simulink library "SLlib_lka_thesis"  (R2018a)
settings: Solver=ode45  StartTime=0.0  StopTime=10.0  RelTol=1e-3  EnableMultiTasking=on
undefined symbols (not defined in the file or in its folder): contr, curvature, DiscIntNeverNeededParam, k, l, pin, sysCtrl
libraries: $bdroot x16, cstblocks x1, simulink x1
(part 1 of 2)
settings Model: Creator=Georg  LastModifiedBy=georgnestlinger
settings DataIOCC: LimitDataPoints=on  SaveFormat=Array  SignalLoggingSaveFormat=ModelDataLogs
settings OptimizationCC: ExpressionDepthLimit=2147483647  LifeSpan=inf
settings DebuggingCC: UnderspecifiedInitializationDetection=Classic  MergeDetectMultiDrivingBlocksExec=none  SolverPrmCheckMsg=warning  FcnCallInpInsideContextMsg=warning  StateNameClashWarn=warning  SFUnexpectedBacktrackingDiag=warning  SFNoUnconditionalDefaultTransitionDiag=warning  SFExecutionAtInitializationDiag=none
settings HardwareCC: ProdBitPerPointer=32  ProdBitPerSizeT=32  ProdBitPerPtrDiffT=32  ProdLargestAtomicFloat=None  ProdIntDivRoundTo=Undefined  ProdEndianess=Unspecified  ProdWordSize=32  ProdHWDeviceType=32-bit Generic
settings ModelReferenceCC: PropagateSignalLabelsOutOfModel=off
settings CodeAppCC: StateflowObjectComments=on
settings GRTTargetCC: TargetLangStandard=C89/C90 (ANSI)  GeneratePreprocessorConditionals=Disable all  CombineOutputUpdateFcns=off  GRTInterface=on
settings ConfigComp: CovMetricSettings=dw  CovHtmlReporting=on  CovSaveCumulativeToWorkspaceVar=on  CovSaveSingleToWorkspaceVar=on  CovExternalEMLEnable=off

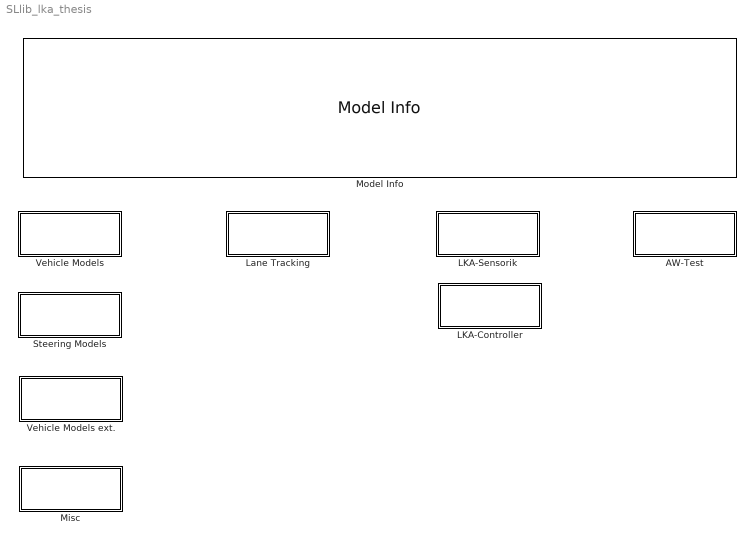
== system SLlib_lka_thesis ==
  AW-Test : Subsystem
  LKA-Controller : Subsystem
  LKA-Sensorik : Subsystem
  Lane Tracking : Subsystem
  Misc : Subsystem
  Model Info : simulink/Model-Wide Utilities/Model Info  Frame=on  DisplayStringWithTags=|  HorizontalTextAlignment=Left  LeftAlignmentValue=0.02
      | Author: Georg Nestlinger
      | Master thesis: Modellbildung und Simulation eines Spurhalteassistenzsystems 
      | 
      | Created: %<Created>
      | 
      | ModifiedBy: %<ModifiedBy>
      | ModifiedComment: %<ModifiedComment>
      | 
      | ModelVersion: %<ModelVersion>
      | ModelName: %<ModelName>
      | 
      | LastModifiedBy: %<LastModifiedBy>
      | LastModidifiedDate: %<LastModificationDate>
  Steering Models : Subsystem
  Vehicle Models : Subsystem
  Vehicle Models ext. : Subsystem

== system SLlib_lka_thesis/AW-Test ==
  AW-Loop : Subsystem
  Plot Interface : Subsystem

== system SLlib_lka_thesis/LKA-Controller ==
  AlgSynth : Subsystem
  FKL : Subsystem
  LKA-Controller : Subsystem  BlockChoice=LQR_2int
      settings: TemplateBlock=self  MemberBlocks=AlgSynth,FKL,LQR,LQR_2int,ZR,ZR_2int
  LQR : Subsystem
  LQR_2int : Subsystem
  State Feedback : Subsystem  TreatAsAtomicUnit=on  mask{fdbk=0}
      mask prompts: fdbk "Feedback parameter:"
  ZR : Subsystem
  ZR_2int : Subsystem

== system SLlib_lka_thesis/LKA-Sensorik ==
  epsL_Sensor : Subsystem
  epsL_exactMdl : Subsystem
  epsL_linMdl : Subsystem
  select epsL : Subsystem  BlockChoice=epsL_Sensor
      settings: TemplateBlock=self  MemberBlocks=epsL_Sensor,epsL_exactMdl,epsL_linMdl
  select yL : Subsystem  BlockChoice=yL_Sensor
      settings: TemplateBlock=self  MemberBlocks=yL_Sensor,yL_exactMdl,yL_linMdl
  yL_Sensor : Subsystem
  yL_exactMdl : Subsystem
  yL_linMdl : Subsystem

== system SLlib_lka_thesis/Lane Tracking ==
  Lane Tracking Model (linear&nonlinear) : Subsystem
  Lane Tracking Model (linear) : Subsystem
  Lane Tracking Model (nonlinear) : Subsystem
  Lane Tracking Sensor : Subsystem

== system SLlib_lka_thesis/Misc ==
  Simout : Subsystem

== system SLlib_lka_thesis/Steering Models ==
  Steering Model (CarMaker DSR) : Subsystem
  Steering Model (CarMaker DSR) [masked] : Subsystem  mask(Steering model parameterization){d_rot=0, d_rack=0, i=0, I_rot=0, m_left=0, m_right=0, m_rack=0, V=0, x0=[0;0]}
      mask prompts: d_rot "d_rot [Nm*s/rad]"; d_rack "d_rack [N*s/rad]"; i "i [rad/m]"; I_rot "I_rot [kg*m²]"; m_left "m_left [kg]"; m_right "m_right [kg]"; m_rack "m_rack [kg]"; V "V [-]"; x0 "Initial value [SWAngle(0); SWRate(0)]"
      mask help:
      | Enter parameters of steering model 'CarMaker Dynamic Steer Ratio'.
      | This model is taken from 'CarMaker Reference Manual, Version 4.0, p. 140'.

== system SLlib_lka_thesis/Vehicle Models ==
  Single Track Models : Subsystem

== system SLlib_lka_thesis/Vehicle Models ext. ==
  Single Track Model (linear) [Initial Values; Interface] : Subsystem
  Single Track Model (linear) [Initial Values; masked] : Subsystem  mask(Linear Single Track Model Inital Values){sy=0, vy=0, yawAngle=0, yawRate=0, x_global=0, y_global=0, s_global=0}
      mask help: Specify initial values for the linear single track model.
  Single Track Model (linear) [Parameter; Interface] : Subsystem
  Single Track Model (linear) [Parameter; masked] : Subsystem  mask(Linear Single Track Model Parameter){cs_front=0, cs_rear=0, l_front=0, l_rear=0, m=0, Izz=0}
      mask prompts: cs_front "Cornering stiffness front [N/rad]"; cs_rear "Cornering stiffness rear [N/rad]"; l_front "Distance COG - front axle [m]"; l_rear "Distance COG - rear axle [m]"; m "Vehicle mass [kg]"; Izz "Moment of inertia of yaw axis [kg*m²]"
      mask help: Specify parameters for the linear single track model.
  Single Track Model/Lane Tracking : Subsystem
  Single Track Model/Lane Tracking/Steering Model : Subsystem
  Single Track Model/Steering Model : Subsystem
  Steering Model (CarMaker DSR) [Parameter; masked] : Subsystem  mask(Steering Model Parameter: Dynamic Steer Ratio){d_rot=0, d_rack=0, i_HR=0, I_rot=0, m_left=0, m_right=0, m_rack=0, V=0, alpha=0}
      mask prompts: d_rot "Damping coefficient of rotating parts [Nm*s/rad]"; d_rack "Damping coefficient of steering rack [Ns/m]"; i_HR "Steering gear ratio steering wheel angle/rack travel [rad/m]"; I_rot "Steering inertia of all rotating parts [kg*m²]"; m_left "Left wheel suspension mass [kg]"; m_right "Right wheel suspension mass [kg]"; m_rack "Steering rack mass [kg]"; V "Amplification of the steering torque [-]"; alpha "Ratio steering wheel angle/front wheel angle [-]"
      mask help: Specify parameters for the CarMaker steering model Dynamic Steer Ratio (DSR).

== system SLlib_lka_thesis/AW-Test/AW-Loop ==
  uPlant : Inport
  delta : Inport  Port=2
  1-D Lookup Table : Lookup_n-D  NumberOfTableDimensions=1  BreakpointsForDimension1=length  Table=curvature  RndMeth=Simplest  InputSameDT=on
  Bus Selector : BusSelector  OutputSignals=vy,yawRate,latOff_LAD_nonlinear,angDev_LAD_nonlinear,SWAngle,SWRate
  Bus Selector1 : BusSelector  OutputSignals=s_global
  Gain2 : Gain  Gain=0
  Regler : Subsystem
  Sum : Sum  Inputs=|-|
  Vehicle Model : Subsystem
  States : Outport
  uCtrl : Outport  Port=2
  wires:
  Vehicle Model/1(VehicleStates) -> Bus Selector1/1, Bus Selector/1, States/1
  Regler/1(u) -> uCtrl/1
  uPlant/1 -> Sum/1
  Bus Selector/1 -> Regler/2(s_yDot)  "<vy>"
  Bus Selector/2 -> Regler/3(psiDot)  "<yawRate>"
  Bus Selector/3 -> Regler/4(yL)  "<latOff_LAD_nonlinear>"
  Bus Selector/4 -> Regler/5(epsL)  "<angDev_LAD_nonlinear>"
  Bus Selector/5 -> Regler/6(steering wheel angle)  "<SWAngle>"
  Bus Selector/6 -> Regler/7(steering wheel angle velocity)  "<SWRate>"
  Sum/1 -> Vehicle Model/1(SWTorque [Nm])
  1-D Lookup Table/1 -> Vehicle Model/3(curvature_LAD [1/m]), Gain2/1
  Bus Selector1/1 -> 1-D Lookup Table/1  "<s_global>"
  Gain2/1 -> Vehicle Model/2(F_left [N])
  delta/1 -> Regler/1(delta)

== system SLlib_lka_thesis/AW-Test/Plot Interface ==
  ideal : Inport
  mit AW : Inport  Port=2
  ohne AW : Inport  Port=3
  Gain : Gain
  Gain1 : Gain
  Gain2 : Gain
  Out1 : Outport
  Out2 : Outport  Port=2
  Out3 : Outport  Port=3
  wires:
  ideal/1 -> Gain/1
  mit AW/1 -> Gain1/1
  ohne AW/1 -> Gain2/1
  Gain/1 -> Out1/1  "ideal"
  Gain1/1 -> Out2/1  "mit AW"
  Gain2/1 -> Out3/1  "ohne AW"

== system SLlib_lka_thesis/LKA-Controller/AlgSynth ==
  r : Inport
  vy : Inport  Port=2
  psiDot : Inport  Port=3
  yL : Inport  Port=4
  epsL : Inport  Port=5
  Controller : Subsystem
  Terminator : Terminator
  Terminator1 : Terminator
  Terminator2 : Terminator
  delta [rad] : Outport
  wires:
  epsL/1 -> Terminator2/1
  vy/1 -> Terminator/1
  psiDot/1 -> Terminator1/1
  yL/1 -> Controller/2(y)
  r/1 -> Controller/1(r)
  Controller/1(u) -> delta [rad]/1

== system SLlib_lka_thesis/LKA-Controller/FKL ==
  r : Inport
  vy : Inport  Port=2
  psiDot : Inport  Port=3
  yL : Inport  Port=4
  epsL : Inport  Port=5
  LTI System R : cstblocks/LTI System  sys=contr.s.AlgSynth.R  IC=[]
  Terminator{1..4} (4 alike) : Terminator
  delta [rad] : Outport
  wires:
  epsL/1 -> Terminator3/1
  vy/1 -> Terminator1/1
  psiDot/1 -> Terminator2/1
  yL/1 -> LTI System R/1
  LTI System R/1 -> delta [rad]/1
  r/1 -> Terminator4/1

== system SLlib_lka_thesis/LKA-Controller/LKA-Controller ==
  r : Inport
  vy : Inport  Port=2
  psiDot : Inport  Port=3
  yL : Inport  Port=4
  epsL : Inport  Port=5
  LQR_2int : $bdroot/LKA-Controller/LQR_2int
  delta [rad] : Outport
  wires:
  r/1 -> LQR_2int/1
  vy/1 -> LQR_2int/2
  psiDot/1 -> LQR_2int/3
  yL/1 -> LQR_2int/4
  epsL/1 -> LQR_2int/5
  LQR_2int/1 -> delta [rad]/1

== system SLlib_lka_thesis/LKA-Controller/LQR ==
  r : Inport
  vy : Inport  Port=2
  psiDot : Inport  Port=3
  yL : Inport  Port=4
  epsL : Inport  Port=5
  Gain1 : Gain  Gain=-contr.t.LQR.k  Multiplication=Matrix(K*u) (u vector)
  Mux : Mux
  Sum1 : Sum  Inputs=-+|
  delta [rad] : Outport
  wires:
  Gain1/1 -> delta [rad]/1
  Mux/1 -> Gain1/1
  epsL/1 -> Mux/4
  vy/1 -> Mux/1
  psiDot/1 -> Mux/2
  yL/1 -> Sum1/2
  Sum1/1 -> Mux/3
  r/1 -> Sum1/1

== system SLlib_lka_thesis/LKA-Controller/LQR_2int ==
  r : Inport
  vy : Inport  Port=2
  psiDot : Inport  Port=3
  yL : Inport  Port=4
  epsL : Inport  Port=5
  Gain : Gain  Gain=-contr.t.LQR_2int.k  Multiplication=Matrix(K*u) (u vector)
  Integrator2 : Integrator
  Integrator3 : Integrator
  Mux2 : Mux  Inputs=6
  Sum1 : Sum  Inputs=-+|
  delta [rad] : Outport
  wires:
  Mux2/1 -> Gain/1
  epsL/1 -> Mux2/4
  vy/1 -> Mux2/1
  psiDot/1 -> Mux2/2
  yL/1 -> Sum1/2
  Sum1/1 -> Mux2/3, Integrator2/1
  r/1 -> Sum1/1
  Integrator2/1 -> Mux2/6, Integrator3/1
  Integrator3/1 -> Mux2/5
  Gain/1 -> delta [rad]/1

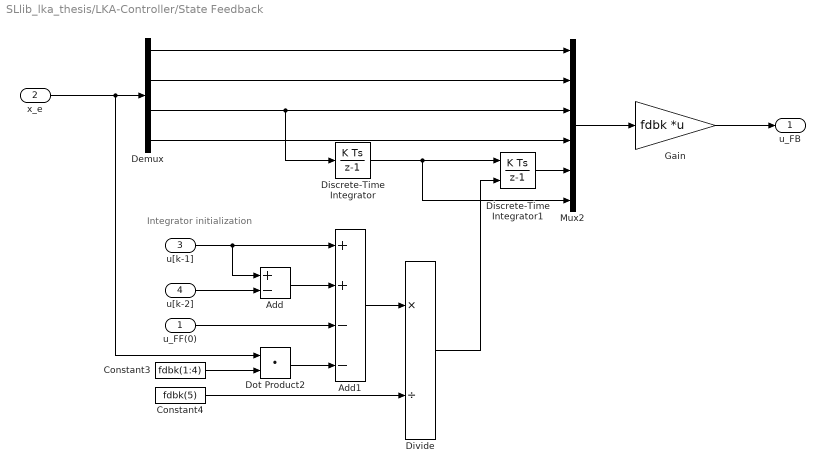
== system SLlib_lka_thesis/LKA-Controller/State Feedback ==
  note: Integrator initialization
  u_FF(0) : Inport
  x_e : Inport  Port=2
  u[k-1] : Inport  Port=3
  u[k-2] : Inport  Port=4
  Add : Sum  Inputs=+-
  Add1 : Sum  Inputs=++--
  Constant3 : Constant  Value=fdbk(1:4)
  Constant4 : Constant  Value=fdbk(5)
  Demux : Demux
  Discrete-Time Integrator : DiscreteIntegrator  SampleTime=-1  ICPrevOutput=DiscIntNeverNeededParam  ICPrevScaledInput=DiscIntNeverNeededParam
  Discrete-Time Integrator1 : DiscreteIntegrator  InitialConditionSource=external  SampleTime=-1  ICPrevOutput=DiscIntNeverNeededParam  ICPrevScaledInput=DiscIntNeverNeededParam
  Divide : Product  Inputs=*/
  Dot Product2 : DotProduct  InputSameDT=on  OutDataTypeStr=Inherit: Inherit via internal rule
  Gain : Gain  Gain=fdbk  Multiplication=Matrix(K*u) (u vector)
  Mux2 : Mux  Inputs=6
  u_FB : Outport
  wires:
  u[k-2]/1 -> Add/2
  Demux/1 -> Mux2/1
  Divide/1 -> Discrete-Time Integrator1/2
  x_e/1 -> Dot Product2/1, Demux/1
  Add1/1 -> Divide/1
  Demux/2 -> Mux2/2
  Mux2/1 -> Gain/1
  u[k-1]/1 -> Add/1, Add1/1
  Demux/3 -> Discrete-Time Integrator/1, Mux2/3
  Constant4/1 -> Divide/2
  Constant3/1 -> Dot Product2/2
  Demux/4 -> Mux2/4
  Discrete-Time Integrator1/1 -> Mux2/5
  Gain/1 -> u_FB/1
  Discrete-Time Integrator/1 -> Discrete-Time Integrator1/1, Mux2/6
  Dot Product2/1 -> Add1/4
  u_FF(0)/1 -> Add1/3
  Add/1 -> Add1/2

== system SLlib_lka_thesis/LKA-Controller/ZR ==
  r : Inport
  vy : Inport  Port=2
  psiDot : Inport  Port=3
  yL : Inport  Port=4
  epsL : Inport  Port=5
  Gain1 : Gain  Gain=-contr.t.ZR.k  Multiplication=Matrix(K*u) (u vector)
  Mux : Mux
  Sum1 : Sum  Inputs=-+|
  delta [rad] : Outport
  wires:
  Gain1/1 -> delta [rad]/1
  Mux/1 -> Gain1/1
  epsL/1 -> Mux/4
  vy/1 -> Mux/1
  psiDot/1 -> Mux/2
  yL/1 -> Sum1/2
  Sum1/1 -> Mux/3
  r/1 -> Sum1/1

== system SLlib_lka_thesis/LKA-Controller/ZR_2int ==
  r : Inport
  vy : Inport  Port=2
  psiDot : Inport  Port=3
  yL : Inport  Port=4
  epsL : Inport  Port=5
  Gain1 : Gain  Gain=-contr.t.ZR_2int.k  Multiplication=Matrix(K*u) (u vector)
  Integrator2 : Integrator
  Integrator3 : Integrator
  Mux2 : Mux  Inputs=6
  Sum1 : Sum  Inputs=-+|
  delta [rad] : Outport
  wires:
  Mux2/1 -> Gain1/1
  epsL/1 -> Mux2/4
  vy/1 -> Mux2/1
  psiDot/1 -> Mux2/2
  yL/1 -> Sum1/2
  Sum1/1 -> Mux2/3, Integrator2/1
  r/1 -> Sum1/1
  Integrator2/1 -> Mux2/6, Integrator3/1
  Integrator3/1 -> Mux2/5
  Gain1/1 -> delta [rad]/1

== system SLlib_lka_thesis/LKA-Sensorik/epsL_Sensor ==
  Vehicle_Data : Inport
  Bus Selector8 : BusSelector  OutputSignals=Sensor.angularDev_LAD_Sensor
  epsL : Outport
  wires:
  Vehicle_Data/1 -> Bus Selector8/1
  Bus Selector8/1 -> epsL/1  "<angularDev_LAD_Sensor>"

== system SLlib_lka_thesis/LKA-Sensorik/epsL_exactMdl ==
  Vehicle_Data : Inport
  Bus Selector8 : BusSelector  OutputSignals=VehicleState.angularDev_LAD_nonlinear
  epsL : Outport
  wires:
  Vehicle_Data/1 -> Bus Selector8/1
  Bus Selector8/1 -> epsL/1  "<angularDev_LAD_nonlinear>"

== system SLlib_lka_thesis/LKA-Sensorik/epsL_linMdl ==
  Vehicle_Data : Inport
  Bus Selector8 : BusSelector  OutputSignals=VehicleState.angularDev_LAD_linear
  epsL : Outport
  wires:
  Vehicle_Data/1 -> Bus Selector8/1
  Bus Selector8/1 -> epsL/1  "<angularDev_LAD_linear>"

== system SLlib_lka_thesis/LKA-Sensorik/select epsL ==
  Vehicle_Data : Inport
  epsL_Sensor : $bdroot/LKA-Sensorik/epsL_Sensor
  epsL : Outport
  wires:
  Vehicle_Data/1 -> epsL_Sensor/1
  epsL_Sensor/1 -> epsL/1

== system SLlib_lka_thesis/LKA-Sensorik/select yL ==
  Vehicle_Data : Inport
  yL_Sensor : $bdroot/LKA-Sensorik/yL_Sensor
  yL : Outport
  wires:
  Vehicle_Data/1 -> yL_Sensor/1
  yL_Sensor/1 -> yL/1

== system SLlib_lka_thesis/LKA-Sensorik/yL_Sensor ==
  Vehicle_Data : Inport
  Bus Selector8 : BusSelector  OutputSignals=Sensor.lateralOff_LAD_Sensor
  yL : Outport
  wires:
  Vehicle_Data/1 -> Bus Selector8/1
  Bus Selector8/1 -> yL/1  "<lateralOff_LAD_Sensor>"

== system SLlib_lka_thesis/LKA-Sensorik/yL_exactMdl ==
  Vehicle_Data : Inport
  Bus Selector8 : BusSelector  OutputSignals=VehicleState.lateralOff_LAD_nonlinear
  yL : Outport
  wires:
  Bus Selector8/1 -> yL/1  "<lateralOff_LAD_nonlinear>"
  Vehicle_Data/1 -> Bus Selector8/1

== system SLlib_lka_thesis/LKA-Sensorik/yL_linMdl ==
  Vehicle_Data : Inport
  Bus Selector1 : BusSelector  OutputSignals=VehicleState.lateralOff_LAD_linear
  yL : Outport
  wires:
  Vehicle_Data/1 -> Bus Selector1/1
  Bus Selector1/1 -> yL/1  "<lateralOff_LAD_linear>"

== system SLlib_lka_thesis/Lane Tracking/Lane Tracking Model (linear&nonlinear) ==
  vx [m/s] : Inport  OutDataTypeStr=double  PortDimensions=1
  vy [m/s] : Inport  Port=2  OutDataTypeStr=double  PortDimensions=1
  yawRate [rad/s] : Inport  Port=3  OutDataTypeStr=double  PortDimensions=1
  LAD [m] : Inport  Port=4  OutDataTypeStr=double  PortDimensions=1
  curvature_LAD [1/m] : Inport  Port=5  OutDataTypeStr=double  PortDimensions=1
  lateralOff_LAD(0) [m] : Inport  Port=6  OutDataTypeStr=double  PortDimensions=1
  angularDev_LAD(0) [rad] : Inport  Port=7  OutDataTypeStr=double  PortDimensions=1
  Bus Creator : BusCreator  Inputs=4
  Lane Tracking Model (linear) : $bdroot/Lane Tracking/Lane Tracking Model (linear)
  Lane Tracking Model (nonlinear) : $bdroot/Lane Tracking/Lane Tracking Model (nonlinear)
  LaneTracking : Outport
  wires:
  vx [m/s]/1 -> Lane Tracking Model (linear)/1, Lane Tracking Model (nonlinear)/1
  vy [m/s]/1 -> Lane Tracking Model (linear)/2, Lane Tracking Model (nonlinear)/2
  yawRate [rad/s]/1 -> Lane Tracking Model (linear)/3, Lane Tracking Model (nonlinear)/3
  LAD [m]/1 -> Lane Tracking Model (linear)/4, Lane Tracking Model (nonlinear)/4
  curvature_LAD [1/m]/1 -> Lane Tracking Model (linear)/5, Lane Tracking Model (nonlinear)/5
  lateralOff_LAD(0) [m]/1 -> Lane Tracking Model (linear)/6, Lane Tracking Model (nonlinear)/6
  angularDev_LAD(0) [rad]/1 -> Lane Tracking Model (linear)/7, Lane Tracking Model (nonlinear)/7
  Bus Creator/1 -> LaneTracking/1  "LaneTracking"
  Lane Tracking Model (linear)/1 -> Bus Creator/1
  Lane Tracking Model (nonlinear)/2 -> Bus Creator/4
  Lane Tracking Model (linear)/2 -> Bus Creator/2
  Lane Tracking Model (nonlinear)/1 -> Bus Creator/3

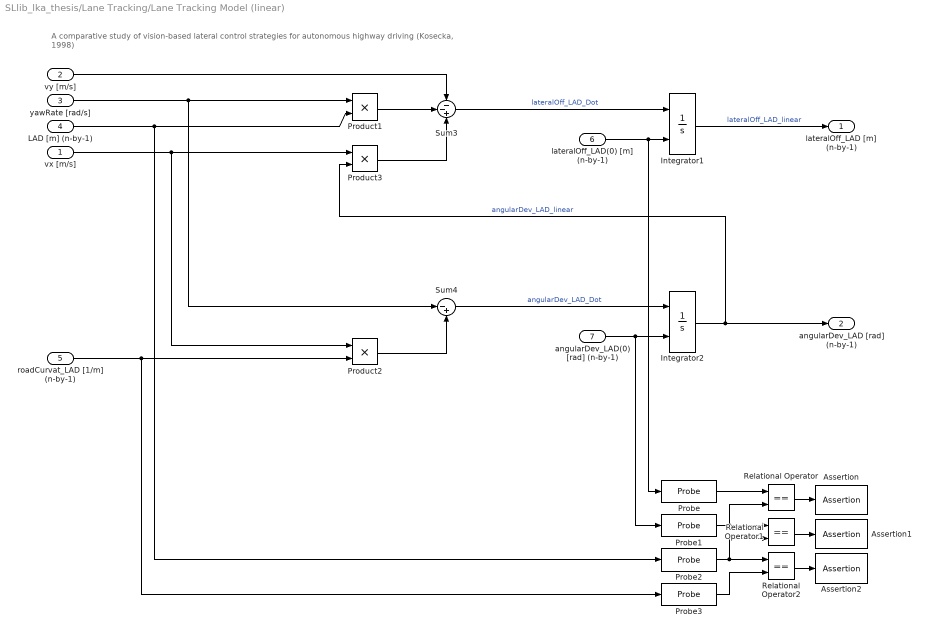
== system SLlib_lka_thesis/Lane Tracking/Lane Tracking Model (linear) ==
  note: A comparative study of vision-based lateral control strategies for autonomous highway driving (Kosecka, 1998)
  vx [m/s] : Inport  OutDataTypeStr=double  Unit=m/s  PortDimensions=1
  vy [m/s] : Inport  Port=2  OutDataTypeStr=double  Unit=m/s  PortDimensions=1
  yawRate [rad/s] : Inport  Port=3  OutDataTypeStr=double  Unit=rad/s  PortDimensions=1
  LAD [m] (n-by-1) : Inport  Port=4  OutDataTypeStr=double  Unit=m
  roadCurvat_LAD [1/m] (n-by-1) : Inport  Port=5  OutDataTypeStr=double  Unit=1/m
  lateralOff_LAD(0) [m] (n-by-1) : Inport  Port=6  OutDataTypeStr=double  Unit=meter
  angularDev_LAD(0) [rad] (n-by-1) : Inport  Port=7  OutDataTypeStr=double  Unit=rad
  Assertion : Assertion
  Assertion1 : Assertion
  Assertion2 : Assertion
  Integrator1 : Integrator  InitialConditionSource=external  InitialCondition=pin.VehicleModel.initialValue.yL
  Integrator2 : Integrator  InitialConditionSource=external  InitialCondition=pin.VehicleModel.initialValue.yL
  Probe{,1..3} (4 alike) : Probe  ProbeWidth=off  ProbeSampleTime=off  ProbeComplexSignal=off  ProbeSignalDimensions=on
  Product1 : Product  RndMeth=Zero
  Product2 : Product  RndMeth=Zero
  Product3 : Product  RndMeth=Zero
  Relational Operator : RelationalOperator  Operator===  OutDataTypeStr=boolean  RndMeth=Nearest
  Relational Operator1 : RelationalOperator  Operator===  OutDataTypeStr=boolean  RndMeth=Nearest
  Relational Operator2 : RelationalOperator  Operator===  OutDataTypeStr=boolean  RndMeth=Nearest
  Sum3 : Sum  Inputs=--+
  Sum4 : Sum  Inputs=|-+
  lateralOff_LAD [m] (n-by-1) : Outport  OutDataTypeStr=double  Unit=m
  angularDev_LAD [rad] (n-by-1) : Outport  Port=2  OutDataTypeStr=double  Unit=rad
  wires:
  roadCurvat_LAD [1/m] (n-by-1)/1 -> Product2/2, Probe3/1
  Integrator1/1 -> lateralOff_LAD [m] (n-by-1)/1  "lateralOff_LAD_linear"
  yawRate [rad/s]/1 -> Product1/1, Sum4/1
  vy [m/s]/1 -> Sum3/1
  Integrator2/1 -> angularDev_LAD [rad] (n-by-1)/1, Product3/2  "angularDev_LAD_linear"
  Product3/1 -> Sum3/3
  Sum3/1 -> Integrator1/1  "lateralOff_LAD_Dot"
  Sum4/1 -> Integrator2/1  "angularDev_LAD_Dot"
  Product2/1 -> Sum4/2
  vx [m/s]/1 -> Product2/1, Product3/1
  LAD [m] (n-by-1)/1 -> Product1/2, Probe2/1
  Product1/1 -> Sum3/2
  angularDev_LAD(0) [rad] (n-by-1)/1 -> Integrator2/2, Probe1/1
  lateralOff_LAD(0) [m] (n-by-1)/1 -> Integrator1/2, Probe/1
  Probe/1 -> Relational Operator/1
  Relational Operator/1 -> Assertion/1
  Relational Operator1/1 -> Assertion1/1
  Relational Operator2/1 -> Assertion2/1
  Probe1/1 -> Relational Operator1/1, Relational Operator/2
  Probe2/1 -> Relational Operator2/1, Relational Operator1/2
  Probe3/1 -> Relational Operator2/2

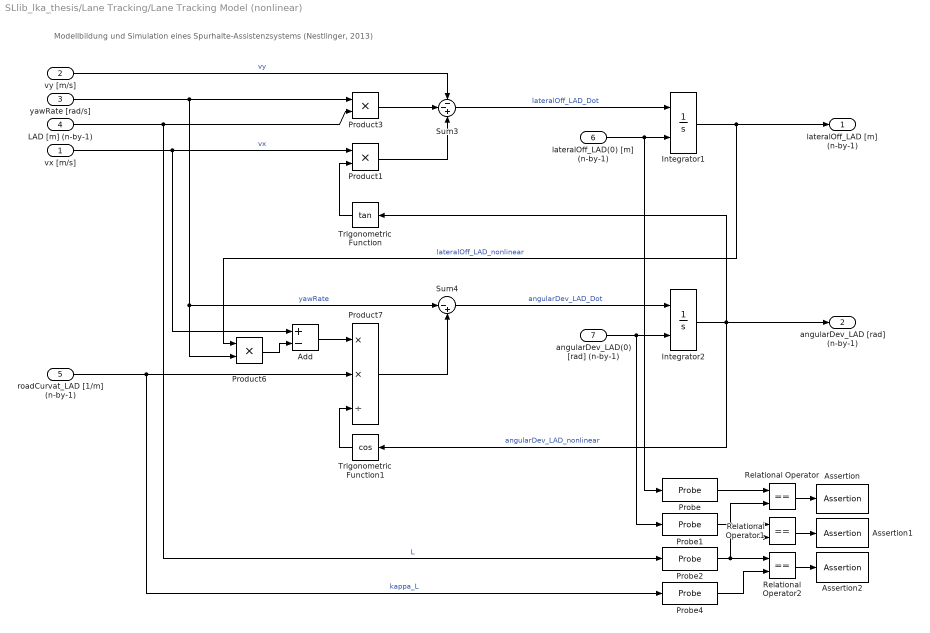
== system SLlib_lka_thesis/Lane Tracking/Lane Tracking Model (nonlinear) ==
  note: Modellbildung und Simulation eines Spurhalte-Assistenzsystems (Nestlinger, 2013)
  vx [m/s] : Inport  OutDataTypeStr=double  PortDimensions=1
  vy [m/s] : Inport  Port=2  OutDataTypeStr=double  PortDimensions=1
  yawRate [rad/s] : Inport  Port=3  OutDataTypeStr=double  PortDimensions=1
  LAD [m] (n-by-1) : Inport  Port=4  OutDataTypeStr=double
  roadCurvat_LAD [1/m] (n-by-1) : Inport  Port=5  OutDataTypeStr=double
  lateralOff_LAD(0) [m] (n-by-1) : Inport  Port=6  OutDataTypeStr=double
  angularDev_LAD(0) [rad] (n-by-1) : Inport  Port=7  OutDataTypeStr=double
  Add : Sum  Inputs=+-
  Assertion : Assertion
  Assertion1 : Assertion
  Assertion2 : Assertion
  Integrator1 : Integrator  InitialConditionSource=external  InitialCondition=pin.VehicleModel.initialValue.yL
  Integrator2 : Integrator  InitialConditionSource=external  InitialCondition=pin.VehicleModel.initialValue.yL
  Probe{,1..2,4} (4 alike) : Probe  ProbeWidth=off  ProbeSampleTime=off  ProbeComplexSignal=off  ProbeSignalDimensions=on
  Product1 : Product  RndMeth=Zero
  Product3 : Product  RndMeth=Zero
  Product6 : Product  RndMeth=Zero
  Product7 : Product  Inputs=**/  RndMeth=Zero
  Relational Operator : RelationalOperator  Operator===  OutDataTypeStr=boolean  RndMeth=Nearest
  Relational Operator1 : RelationalOperator  Operator===  OutDataTypeStr=boolean  RndMeth=Nearest
  Relational Operator2 : RelationalOperator  Operator===  OutDataTypeStr=boolean  RndMeth=Nearest
  Sum3 : Sum  Inputs=--+
  Sum4 : Sum  Inputs=|-+
  Trigonometric Function : Trigonometry  Operator=tan
  Trigonometric Function1 : Trigonometry  Operator=cos
  lateralOff_LAD [m] (n-by-1) : Outport  OutDataTypeStr=double
  angularDev_LAD [rad] (n-by-1) : Outport  Port=2  OutDataTypeStr=double
  wires:
  Product7/1 -> Sum4/2
  angularDev_LAD(0) [rad] (n-by-1)/1 -> Integrator2/2, Probe1/1
  lateralOff_LAD(0) [m] (n-by-1)/1 -> Integrator1/2, Probe/1
  Trigonometric Function1/1 -> Product7/3
  roadCurvat_LAD [1/m] (n-by-1)/1 -> Probe4/1, Product7/2  "kappa_L"
  LAD [m] (n-by-1)/1 -> Product3/2, Probe2/1  "L"
  Trigonometric Function/1 -> Product1/2
  vx [m/s]/1 -> Product1/1, Add/1  "vx"
  Product3/1 -> Sum3/2
  Integrator1/1 -> Product6/1, lateralOff_LAD [m] (n-by-1)/1  "lateralOff_LAD_nonlinear"
  yawRate [rad/s]/1 -> Product3/1, Product6/2, Sum4/1  "yawRate"
  vy [m/s]/1 -> Sum3/1  "vy"
  Integrator2/1 -> Trigonometric Function1/1, Trigonometric Function/1, angularDev_LAD [rad] (n-by-1)/1  "angularDev_LAD_nonlinear"
  Product1/1 -> Sum3/3
  Sum3/1 -> Integrator1/1  "lateralOff_LAD_Dot"
  Sum4/1 -> Integrator2/1  "angularDev_LAD_Dot"
  Product6/1 -> Add/2
  Add/1 -> Product7/1
  Probe/1 -> Relational Operator/1
  Relational Operator/1 -> Assertion/1
  Relational Operator1/1 -> Assertion1/1
  Relational Operator2/1 -> Assertion2/1
  Probe1/1 -> Relational Operator1/1, Relational Operator/2
  Probe2/1 -> Relational Operator2/1, Relational Operator1/2
  Probe4/1 -> Relational Operator2/2

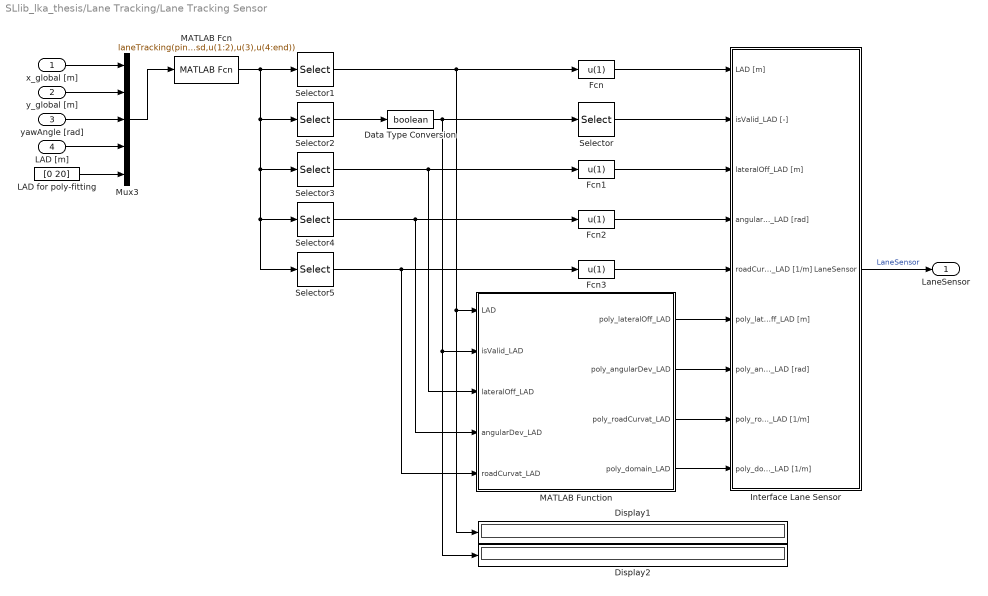
== system SLlib_lka_thesis/Lane Tracking/Lane Tracking Sensor ==
  x_global [m] : Inport  OutDataTypeStr=double  PortDimensions=1
  y_global [m] : Inport  Port=2  OutDataTypeStr=double  PortDimensions=1
  yawAngle [rad] : Inport  Port=3  OutDataTypeStr=double  PortDimensions=1
  LAD [m] : Inport  Port=4  OutDataTypeStr=double  PortDimensions=1
  Data Type Conversion : DataTypeConversion  OutDataTypeStr=boolean
  Display1 : Display
  Display2 : Display
  Fcn{,1..3} (4 alike) : Fcn  Expr=u(1)
  Interface Lane Sensor : Subsystem
  LAD for poly-fitting : Constant  Value=[0 20]
  MATLAB Fcn : MATLABFcn  MATLABFcn=laneTracking(pin.traj_sd,u(1:2),u(3),u(4:end))  Output1D=off
  MATLAB Function : MATLAB Function  TreatAsAtomicUnit=on
  Mux3 : Mux  Inputs=5
  Selector : Selector  NumberOfDimensions=2  InputPortWidth=1  IndexOptions=Index vector (dialog),Index vector (dialog)  Indices=1,1  OutputSizes=1,1
  Selector1 : Selector  NumberOfDimensions=2  InputPortWidth=3  IndexOptions=Index vector (dialog),Select all  Indices=1,1  OutputSizes=1,3
  Selector2 : Selector  NumberOfDimensions=2  InputPortWidth=3  IndexOptions=Index vector (dialog),Select all  Indices=2,1  OutputSizes=1,3
  Selector3 : Selector  NumberOfDimensions=2  InputPortWidth=3  IndexOptions=Index vector (dialog),Select all  Indices=3,1  OutputSizes=1,3
  Selector4 : Selector  NumberOfDimensions=2  InputPortWidth=3  IndexOptions=Index vector (dialog),Select all  Indices=4,1  OutputSizes=1,3
  Selector5 : Selector  NumberOfDimensions=2  InputPortWidth=3  IndexOptions=Index vector (dialog),Select all  Indices=5,1  OutputSizes=1,3
  LaneSensor : Outport
  wires:
  MATLAB Function/4(poly_domain_LAD) -> Interface Lane Sensor/9(poly_domain_LAD [1/m])
  Fcn3/1 -> Interface Lane Sensor/5(roadCurv_LAD [1/m])
  Fcn2/1 -> Interface Lane Sensor/4(angularDev_LAD [rad])
  Fcn1/1 -> Interface Lane Sensor/3(lateralOff_LAD [m])
  Selector/1 -> Interface Lane Sensor/2(isValid_LAD [-])
  Fcn/1 -> Interface Lane Sensor/1(LAD [m])
  LAD [m]/1 -> Mux3/4
  LAD for poly-fitting/1 -> Mux3/5
  MATLAB Function/3(poly_roadCurvat_LAD) -> Interface Lane Sensor/8(poly_roadCurvat_LAD [1/m])
  MATLAB Function/2(poly_angularDev_LAD) -> Interface Lane Sensor/7(poly_angularDev_LAD [rad])
  MATLAB Function/1(poly_lateralOff_LAD) -> Interface Lane Sensor/6(poly_lateralOff_LAD [m])
  Data Type Conversion/1 -> Display2/1, MATLAB Function/2(isValid_LAD), Selector/1
  Selector5/1 -> Fcn3/1, MATLAB Function/5(roadCurvat_LAD)
  Selector4/1 -> Fcn2/1, MATLAB Function/4(angularDev_LAD)
  Selector3/1 -> Fcn1/1, MATLAB Function/3(lateralOff_LAD)
  Selector2/1 -> Data Type Conversion/1
  Selector1/1 -> Display1/1, MATLAB Function/1(LAD), Fcn/1
  MATLAB Fcn/1 -> Selector1/1, Selector2/1, Selector3/1, Selector5/1, Selector4/1
  x_global [m]/1 -> Mux3/1
  Mux3/1 -> MATLAB Fcn/1
  yawAngle [rad]/1 -> Mux3/3
  y_global [m]/1 -> Mux3/2
  Interface Lane Sensor/1(LaneSensor) -> LaneSensor/1  "LaneSensor"

== system SLlib_lka_thesis/Misc/Simout ==
  VhclState : Inport
  Control_Input : Inport  Port=2
  LaneTracking : Inport  Port=3
  LaneSensor : Inport  Port=4
  Bus Creator : BusCreator  Inputs=4
  To Workspace : ToWorkspace  VariableName=simout  SaveFormat=Timeseries  SampleTime=-1
  wires:
  LaneTracking/1 -> Bus Creator/4  "LaneTracking"
  VhclState/1 -> Bus Creator/1  "VhclState"
  LaneSensor/1 -> Bus Creator/2  "LaneSensor"
  Control_Input/1 -> Bus Creator/3  "Control"
  Bus Creator/1 -> To Workspace/1

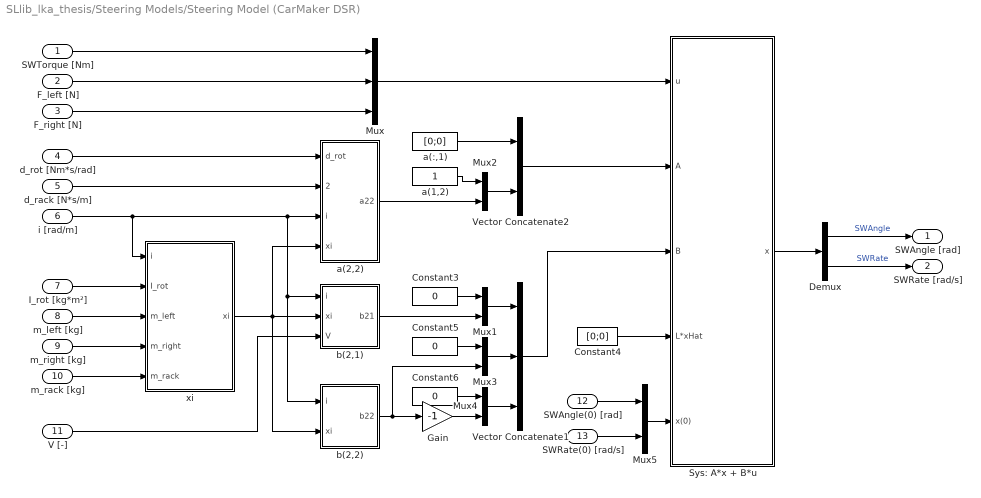
== system SLlib_lka_thesis/Steering Models/Steering Model (CarMaker DSR) ==
  SWTorque [Nm] : Inport  OutDataTypeStr=double  PortDimensions=1
  F_left [N] : Inport  Port=2  OutDataTypeStr=double  PortDimensions=1
  F_right [N] : Inport  Port=3  OutDataTypeStr=double  PortDimensions=1
  d_rot [Nm*s/rad] : Inport  Port=4  OutDataTypeStr=double  PortDimensions=1
  d_rack [N*s/m] : Inport  Port=5  OutDataTypeStr=double  PortDimensions=1
  i [rad/m] : Inport  Port=6  OutDataTypeStr=double  PortDimensions=1
  I_rot [kg*m²] : Inport  Port=7  OutDataTypeStr=double  PortDimensions=1
  m_left [kg] : Inport  Port=8  OutDataTypeStr=double  PortDimensions=1
  m_right [kg] : Inport  Port=9  OutDataTypeStr=double  PortDimensions=1
  m_rack [kg] : Inport  Port=10  OutDataTypeStr=double  PortDimensions=1
  V [-] : Inport  Port=11
  SWAngle(0) [rad] : Inport  Port=12  OutDataTypeStr=double  PortDimensions=1
  SWRate(0) [rad/s] : Inport  Port=13  OutDataTypeStr=double  PortDimensions=1
  Constant3 : Constant  Value=0
  Constant4 : Constant  Value=[0;0]
  Constant5 : Constant  Value=0
  Constant6 : Constant  Value=0
  Demux : Demux  Outputs=2
  Gain : Gain  Gain=-1
  Mux : Mux  Inputs=3
  Mux{1..5} (5 alike) : Mux  Inputs=2
  Sys: A*x + B*u : Subsystem
  Vector Concatenate1 : Concatenate  NumInputs=3  Mode=Multidimensional array  ConcatenateDimension=2
  Vector Concatenate2 : Concatenate  Mode=Multidimensional array  ConcatenateDimension=2
  a(1,2) : Constant
  a(2,2) : Subsystem
  a(:,1) : Constant  Value=[0;0]
  b(2,1) : Subsystem
  b(2,2) : Subsystem
  xi : Subsystem
  SWAngle [rad] : Outport  OutDataTypeStr=double  PortDimensions=1
  SWRate [rad/s] : Outport  Port=2  OutDataTypeStr=double  PortDimensions=1
  wires:
  Vector Concatenate1/1 -> Sys: A*x + B*u/3(B)
  a(1,2)/1 -> Mux2/1
  Mux2/1 -> Vector Concatenate2/2
  a(:,1)/1 -> Vector Concatenate2/1
  Sys: A*x + B*u/1(x) -> Demux/1
  b(2,2)/1(b22) -> Gain/1, Mux3/2
  Vector Concatenate2/1 -> Sys: A*x + B*u/2(A)
  V [-]/1 -> b(2,1)/3(V)
  Demux/2 -> SWRate [rad/s]/1  "SWRate"
  Demux/1 -> SWAngle [rad]/1  "SWAngle"
  F_right [N]/1 -> Mux/3
  F_left [N]/1 -> Mux/2
  SWTorque [Nm]/1 -> Mux/1
  Mux/1 -> Sys: A*x + B*u/1(u)
  xi/1(xi) -> b(2,2)/2(xi), a(2,2)/4(xi), b(2,1)/2(xi)
  a(2,2)/1(a22) -> Mux2/2
  m_right [kg]/1 -> xi/4(m_right)
  m_left [kg]/1 -> xi/3(m_left)
  m_rack [kg]/1 -> xi/5(m_rack)
  d_rack [N*s/m]/1 -> a(2,2)/2(d_rack)
  i [rad/m]/1 -> xi/1(i), b(2,2)/1(i), b(2,1)/1(i), a(2,2)/3(i)
  d_rot [Nm*s/rad]/1 -> a(2,2)/1(d_rot)
  Constant4/1 -> Sys: A*x + B*u/4(L*xHat)
  b(2,1)/1(b21) -> Mux1/2
  Constant3/1 -> Mux1/1
  Mux1/1 -> Vector Concatenate1/1
  Mux3/1 -> Vector Concatenate1/2
  Mux4/1 -> Vector Concatenate1/3
  Constant5/1 -> Mux3/1
  Constant6/1 -> Mux4/1
  Gain/1 -> Mux4/2
  I_rot [kg*m²]/1 -> xi/2(I_rot)
  Mux5/1 -> Sys: A*x + B*u/5(x(0))
  SWAngle(0) [rad]/1 -> Mux5/1
  SWRate(0) [rad/s]/1 -> Mux5/2

== system SLlib_lka_thesis/Steering Models/Steering Model (CarMaker DSR) [masked] ==
  SWTorque [Nm] : Inport
  F_left [N] : Inport  Port=2
  F_right [N] : Inport  Port=3
  Constant : Constant  Value=d_rot
  Constant1 : Constant  Value=d_rack
  Constant2 : Constant  Value=i
  Constant3 : Constant  Value=I_rot
  Constant4 : Constant  Value=m_left
  Constant5 : Constant  Value=m_right
  Constant6 : Constant  Value=m_rack
  Constant7 : Constant  Value=V
  Constant8 : Constant  Value=x0
  Demux : Demux  Outputs=2
  Steering Model (CarMaker DSR) : $bdroot/Steering Models/Steering Model (CarMaker DSR)
  SWAngle [rad] : Outport
  SWRate [rad/s] : Outport  Port=2
  wires:
  Steering Model (CarMaker DSR)/1 -> SWAngle [rad]/1
  Steering Model (CarMaker DSR)/2 -> SWRate [rad/s]/1
  SWTorque [Nm]/1 -> Steering Model (CarMaker DSR)/1
  F_left [N]/1 -> Steering Model (CarMaker DSR)/2
  F_right [N]/1 -> Steering Model (CarMaker DSR)/3
  Constant/1 -> Steering Model (CarMaker DSR)/4
  Constant1/1 -> Steering Model (CarMaker DSR)/5
  Constant2/1 -> Steering Model (CarMaker DSR)/6
  Constant3/1 -> Steering Model (CarMaker DSR)/7
  Constant4/1 -> Steering Model (CarMaker DSR)/8
  Constant5/1 -> Steering Model (CarMaker DSR)/9
  Constant6/1 -> Steering Model (CarMaker DSR)/10
  Constant7/1 -> Steering Model (CarMaker DSR)/11
  Constant8/1 -> Demux/1
  Demux/1 -> Steering Model (CarMaker DSR)/12
  Demux/2 -> Steering Model (CarMaker DSR)/13

== system SLlib_lka_thesis/Vehicle Models/Single Track Models ==
  Single Track Model (linear) : Subsystem
  Single Track Model (linear) [masked] : Subsystem  mask(Linear Single Track Model){cs_front_rear=[0;0], l_front_rear=[0;0], m=0, Izz=0, vx=0, sy_init=0, vy_init=0, yawAngle_init=0, yawRate_init=0, xys_global_init=[0 0 0]}
      mask prompts: cs_front_rear "Cornering stiffness [N/rad]: [cs_front;cs_rear]"; l_front_rear "Distance COG - front/rear axle [m]: [l_front;l_rear]"; m "Vehicle mass [kg]"; Izz "Moment of inertia of yaw axis [kg*m²]"; vx "Longitudinal velocity [m/s]"; sy_init "Initial value sy [m]"; vy_init "Initial value vy [m/s]"; yawAngle_init "Initial value yawAngle [rad]"; yawRate_init "Initial value yawRate [rad/s]"; xys_global_init "Initial position [m]: [x_global;y_global;s_global]"
      mask help: Specify parameters for the linear single track model.

== system SLlib_lka_thesis/Vehicle Models ext./Single Track Model (linear) [Initial Values; Interface] ==
  sy(0) [m] : Inport  OutDataTypeStr=double  PortDimensions=1
  vy(0) [m/s] : Inport  Port=2  OutDataTypeStr=double  PortDimensions=1
  yawAngle(0) [rad] : Inport  Port=3  OutDataTypeStr=double  PortDimensions=1
  yawRate(0) [rad/s] : Inport  Port=4  OutDataTypeStr=double  PortDimensions=1
  x_global(0) [m] : Inport  Port=5  OutDataTypeStr=double  PortDimensions=1
  y_global(0) [m] : Inport  Port=6  OutDataTypeStr=double  PortDimensions=1
  s_global(0) [m] : Inport  Port=7  OutDataTypeStr=double  PortDimensions=1
  Mux : Mux  Inputs=7
  Vhcl_InitValues : Outport
  wires:
  Mux/1 -> Vhcl_InitValues/1
  sy(0) [m]/1 -> Mux/1
  yawRate(0) [rad/s]/1 -> Mux/4
  x_global(0) [m]/1 -> Mux/5
  y_global(0) [m]/1 -> Mux/6
  s_global(0) [m]/1 -> Mux/7
  vy(0) [m/s]/1 -> Mux/2
  yawAngle(0) [rad]/1 -> Mux/3

== system SLlib_lka_thesis/Vehicle Models ext./Single Track Model (linear) [Initial Values; masked] ==
  Constant10 : Constant  Value=y_global
  Constant12 : Constant  Value=s_global
  Constant5 : Constant  Value=sy
  Constant6 : Constant  Value=vy
  Constant7 : Constant  Value=yawAngle
  Constant8 : Constant  Value=yawRate
  Constant9 : Constant  Value=x_global
  Mux : Mux  Inputs=7
  Vhcl_InitValues : Outport
  wires:
  Mux/1 -> Vhcl_InitValues/1
  Constant5/1 -> Mux/1
  Constant6/1 -> Mux/2
  Constant7/1 -> Mux/3
  Constant8/1 -> Mux/4
  Constant9/1 -> Mux/5
  Constant10/1 -> Mux/6
  Constant12/1 -> Mux/7

== system SLlib_lka_thesis/Vehicle Models ext./Single Track Model (linear) [Parameter; Interface] ==
  cs_front [N/rad] : Inport  OutDataTypeStr=double  PortDimensions=1
  cs_rear [N/rad] : Inport  Port=2  OutDataTypeStr=double  PortDimensions=1
  l_front [m] : Inport  Port=3  OutMin=0  OutDataTypeStr=double  PortDimensions=1
  l_rear [m] : Inport  Port=4  OutMin=0  OutDataTypeStr=double  PortDimensions=1
  m [kg] : Inport  Port=5  OutMin=0  OutDataTypeStr=double  PortDimensions=1
  Izz [kg*m²] : Inport  Port=6  OutMin=0  OutDataTypeStr=double  PortDimensions=1
  Bus Creator : BusCreator  Inputs=6
  Vhcl_Parameter : Outport
  wires:
  Izz [kg*m²]/1 -> Bus Creator/6  "Izz"
  m [kg]/1 -> Bus Creator/5  "m"
  l_rear [m]/1 -> Bus Creator/4  "l_rear"
  l_front [m]/1 -> Bus Creator/3  "l_front"
  cs_rear [N/rad]/1 -> Bus Creator/2  "cs_rear"
  cs_front [N/rad]/1 -> Bus Creator/1  "cs_front"
  Bus Creator/1 -> Vhcl_Parameter/1

== system SLlib_lka_thesis/Vehicle Models ext./Single Track Model (linear) [Parameter; masked] ==
  Bus Creator : BusCreator  Inputs=6
  Constant : Constant  Value=cs_front
  Constant1 : Constant  Value=cs_rear
  Constant2 : Constant  Value=l_front
  Constant3 : Constant  Value=l_rear
  Constant4 : Constant  Value=m
  Constant5 : Constant  Value=Izz
  Vhcl_Parameter : Outport
  wires:
  Constant5/1 -> Bus Creator/6  "Izz"
  Constant4/1 -> Bus Creator/5  "m"
  Constant3/1 -> Bus Creator/4  "l_rear"
  Constant2/1 -> Bus Creator/3  "l_front"
  Constant1/1 -> Bus Creator/2  "cs_rear"
  Constant/1 -> Bus Creator/1  "cs_front"
  Bus Creator/1 -> Vhcl_Parameter/1

== system SLlib_lka_thesis/Vehicle Models ext./Single Track Model//Lane Tracking ==
  steerAngle [rad] : Inport
  Vhcl_Parameter : Inport  Port=2
  vx [m/s] : Inport  Port=3
  LAD [m] : Inport  Port=4
  curvature_LAD [1/m] : Inport  Port=5
  latOff_LAD(0) [m] : Inport  Port=6
  angDev_LAD(0) [rad] : Inport  Port=7
  Vhcl_InitValues : Inport  Port=8
  Bus Creator1 : BusCreator  Inputs=11
  Bus Selector1 : BusSelector  OutputSignals=cs_front,cs_rear,l_front,l_rear,m,Izz
  Demux : Demux  Outputs=7
  Lane Tracking Model (linear) : $bdroot/Lane Tracking/Lane Tracking Model (linear)
  Lane Tracking Model (nonlinear) : $bdroot/Lane Tracking/Lane Tracking Model (nonlinear)
  Single Track Model (linear) : $bdroot/Vehicle Models/Single Track Models/Single Track Model (linear)
  VehicleState : Outport
  wires:
  curvature_LAD [1/m]/1 -> Lane Tracking Model (linear)/5, Lane Tracking Model (nonlinear)/5
  Bus Creator1/1 -> VehicleState/1  "VehicleState"
  Single Track Model (linear)/1 -> Bus Creator1/1
  Single Track Model (linear)/2 -> Bus Creator1/2, Lane Tracking Model (linear)/2, Lane Tracking Model (nonlinear)/2
  Single Track Model (linear)/4 -> Bus Creator1/4, Lane Tracking Model (linear)/3, Lane Tracking Model (nonlinear)/3
  Lane Tracking Model (linear)/1 -> Bus Creator1/8
  Lane Tracking Model (linear)/2 -> Bus Creator1/9
  Lane Tracking Model (nonlinear)/1 -> Bus Creator1/10
  Lane Tracking Model (nonlinear)/2 -> Bus Creator1/11
  angDev_LAD(0) [rad]/1 -> Lane Tracking Model (linear)/7, Lane Tracking Model (nonlinear)/7
  latOff_LAD(0) [m]/1 -> Lane Tracking Model (linear)/6, Lane Tracking Model (nonlinear)/6
  LAD [m]/1 -> Lane Tracking Model (linear)/4, Lane Tracking Model (nonlinear)/4
  vx [m/s]/1 -> Lane Tracking Model (linear)/1, Lane Tracking Model (nonlinear)/1, Single Track Model (linear)/8
  Vhcl_Parameter/1 -> Bus Selector1/1
  Single Track Model (linear)/3 -> Bus Creator1/3
  Single Track Model (linear)/7 -> Bus Creator1/7
  Single Track Model (linear)/6 -> Bus Creator1/6
  Single Track Model (linear)/5 -> Bus Creator1/5
  Bus Selector1/6 -> Single Track Model (linear)/7  "<Izz>"
  Bus Selector1/5 -> Single Track Model (linear)/6  "<m>"
  Bus Selector1/4 -> Single Track Model (linear)/5  "<l_rear>"
  Bus Selector1/3 -> Single Track Model (linear)/4  "<l_front>"
  Bus Selector1/2 -> Single Track Model (linear)/3  "<cs_rear>"
  Bus Selector1/1 -> Single Track Model (linear)/2  "<cs_front>"
  steerAngle [rad]/1 -> Single Track Model (linear)/1
  Vhcl_InitValues/1 -> Demux/1
  Demux/1 -> Single Track Model (linear)/9
  Demux/2 -> Single Track Model (linear)/10
  Demux/3 -> Single Track Model (linear)/11
  Demux/4 -> Single Track Model (linear)/12
  Demux/5 -> Single Track Model (linear)/13
  Demux/6 -> Single Track Model (linear)/14
  Demux/7 -> Single Track Model (linear)/15

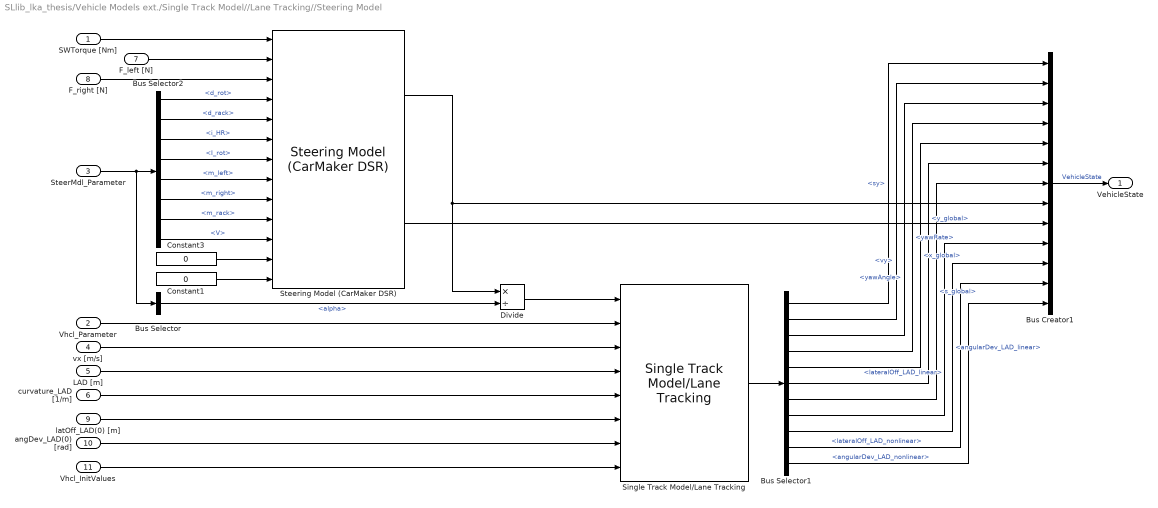
== system SLlib_lka_thesis/Vehicle Models ext./Single Track Model//Lane Tracking//Steering Model ==
  SWTorque [Nm] : Inport
  Vhcl_Parameter : Inport  Port=2
  SteerMdl_Parameter : Inport  Port=3
  vx [m/s] : Inport  Port=4
  LAD [m] : Inport  Port=5
  curvature_LAD [1/m] : Inport  Port=6
  F_left [N] : Inport  Port=7
  F_right [N] : Inport  Port=8
  latOff_LAD(0) [m] : Inport  Port=9
  angDev_LAD(0) [rad] : Inport  Port=10
  Vhcl_InitValues : Inport  Port=11
  Bus Creator1 : BusCreator  Inputs=13
  Bus Selector : BusSelector  OutputSignals=alpha
  Bus Selector1 : BusSelector  OutputSignals=sy,vy,yawAngle,yawRate,x_global,y_global,s_global,lateralOff_LAD_linear,angularDev_LAD_linear,lateralOff_LAD_nonlinear,angularDev_LAD_nonlinear
  Bus Selector2 : BusSelector  OutputSignals=d_rot,d_rack,i_HR,I_rot,m_left,m_right,m_rack,V
  Constant1 : Constant  Value=0
  Constant3 : Constant  Value=0
  Divide : Product  Inputs=*/
  Single Track Model/Lane Tracking : $bdroot/Vehicle Models ext./Single Track Model//Lane Tracking
  Steering Model (CarMaker DSR) : $bdroot/Steering Models/Steering Model (CarMaker DSR)
  VehicleState : Outport
  wires:
  Bus Selector/1 -> Divide/2  "<alpha>"
  angDev_LAD(0) [rad]/1 -> Single Track Model/Lane Tracking/7
  SWTorque [Nm]/1 -> Steering Model (CarMaker DSR)/1
  Steering Model (CarMaker DSR)/1 -> Bus Creator1/8, Divide/1
  Vhcl_Parameter/1 -> Single Track Model/Lane Tracking/2
  vx [m/s]/1 -> Single Track Model/Lane Tracking/3
  LAD [m]/1 -> Single Track Model/Lane Tracking/4
  latOff_LAD(0) [m]/1 -> Single Track Model/Lane Tracking/6
  Bus Creator1/1 -> VehicleState/1  "VehicleState"
  curvature_LAD [1/m]/1 -> Single Track Model/Lane Tracking/5
  SteerMdl_Parameter/1 -> Bus Selector/1, Bus Selector2/1
  Divide/1 -> Single Track Model/Lane Tracking/1
  Steering Model (CarMaker DSR)/2 -> Bus Creator1/9
  Single Track Model/Lane Tracking/1 -> Bus Selector1/1
  Vhcl_InitValues/1 -> Single Track Model/Lane Tracking/8
  Bus Selector1/1 -> Bus Creator1/1  "<sy>"
  Bus Selector1/2 -> Bus Creator1/2  "<vy>"
  Bus Selector1/3 -> Bus Creator1/3  "<yawAngle>"
  Bus Selector1/4 -> Bus Creator1/4  "<yawRate>"
  Bus Selector1/5 -> Bus Creator1/5  "<x_global>"
  Bus Selector1/6 -> Bus Creator1/6  "<y_global>"
  Bus Selector1/7 -> Bus Creator1/7  "<s_global>"
  Bus Selector1/8 -> Bus Creator1/10  "<lateralOff_LAD_linear>"
  Bus Selector1/9 -> Bus Creator1/11  "<angularDev_LAD_linear>"
  Bus Selector1/10 -> Bus Creator1/12  "<lateralOff_LAD_nonlinear>"
  Bus Selector1/11 -> Bus Creator1/13  "<angularDev_LAD_nonlinear>"
  F_left [N]/1 -> Steering Model (CarMaker DSR)/2
  F_right [N]/1 -> Steering Model (CarMaker DSR)/3
  Bus Selector2/1 -> Steering Model (CarMaker DSR)/4  "<d_rot>"
  Bus Selector2/2 -> Steering Model (CarMaker DSR)/5  "<d_rack>"
  Bus Selector2/3 -> Steering Model (CarMaker DSR)/6  "<i_HR>"
  Bus Selector2/4 -> Steering Model (CarMaker DSR)/7  "<I_rot>"
  Bus Selector2/5 -> Steering Model (CarMaker DSR)/8  "<m_left>"
  Bus Selector2/6 -> Steering Model (CarMaker DSR)/9  "<m_right>"
  Bus Selector2/7 -> Steering Model (CarMaker DSR)/10  "<m_rack>"
  Bus Selector2/8 -> Steering Model (CarMaker DSR)/11  "<V>"
  Constant3/1 -> Steering Model (CarMaker DSR)/12
  Constant1/1 -> Steering Model (CarMaker DSR)/13

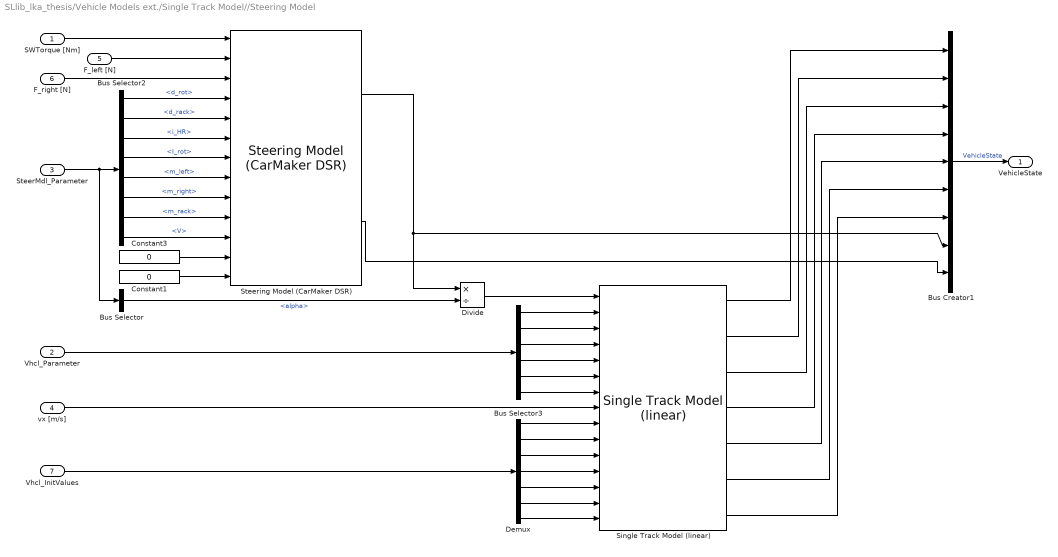
== system SLlib_lka_thesis/Vehicle Models ext./Single Track Model//Steering Model ==
  SWTorque [Nm] : Inport
  Vhcl_Parameter : Inport  Port=2
  SteerMdl_Parameter : Inport  Port=3
  vx [m/s] : Inport  Port=4
  F_left [N] : Inport  Port=5
  F_right [N] : Inport  Port=6
  Vhcl_InitValues : Inport  Port=7
  Bus Creator1 : BusCreator  Inputs=9
  Bus Selector : BusSelector  OutputSignals=alpha
  Bus Selector2 : BusSelector  OutputSignals=d_rot,d_rack,i_HR,I_rot,m_left,m_right,m_rack,V
  Bus Selector3 : BusSelector  OutputSignals=cs_front,cs_rear,l_front,l_rear,m,Izz
  Constant1 : Constant  Value=0
  Constant3 : Constant  Value=0
  Demux : Demux  Outputs=7
  Divide : Product  Inputs=*/
  Single Track Model (linear) : $bdroot/Vehicle Models/Single Track Models/Single Track Model (linear)
  Steering Model (CarMaker DSR) : $bdroot/Steering Models/Steering Model (CarMaker DSR)
  VehicleState : Outport
  wires:
  Vhcl_InitValues/1 -> Demux/1
  Constant1/1 -> Steering Model (CarMaker DSR)/13
  Constant3/1 -> Steering Model (CarMaker DSR)/12
  Bus Selector2/8 -> Steering Model (CarMaker DSR)/11  "<V>"
  Bus Selector2/7 -> Steering Model (CarMaker DSR)/10  "<m_rack>"
  Bus Selector2/6 -> Steering Model (CarMaker DSR)/9  "<m_right>"
  Bus Selector2/5 -> Steering Model (CarMaker DSR)/8  "<m_left>"
  Bus Selector2/4 -> Steering Model (CarMaker DSR)/7  "<I_rot>"
  Bus Selector2/3 -> Steering Model (CarMaker DSR)/6  "<i_HR>"
  Bus Selector2/2 -> Steering Model (CarMaker DSR)/5  "<d_rack>"
  Bus Selector2/1 -> Steering Model (CarMaker DSR)/4  "<d_rot>"
  F_right [N]/1 -> Steering Model (CarMaker DSR)/3
  F_left [N]/1 -> Steering Model (CarMaker DSR)/2
  Single Track Model (linear)/7 -> Bus Creator1/7
  Single Track Model (linear)/6 -> Bus Creator1/6
  Single Track Model (linear)/5 -> Bus Creator1/5
  Single Track Model (linear)/4 -> Bus Creator1/4
  Single Track Model (linear)/3 -> Bus Creator1/3
  Single Track Model (linear)/2 -> Bus Creator1/2
  Single Track Model (linear)/1 -> Bus Creator1/1
  Steering Model (CarMaker DSR)/2 -> Bus Creator1/9
  Divide/1 -> Single Track Model (linear)/1
  SteerMdl_Parameter/1 -> Bus Selector2/1, Bus Selector/1
  Bus Creator1/1 -> VehicleState/1  "VehicleState"
  vx [m/s]/1 -> Single Track Model (linear)/8
  Vhcl_Parameter/1 -> Bus Selector3/1
  Steering Model (CarMaker DSR)/1 -> Divide/1, Bus Creator1/8
  SWTorque [Nm]/1 -> Steering Model (CarMaker DSR)/1
  Bus Selector/1 -> Divide/2  "<alpha>"
  Bus Selector3/1 -> Single Track Model (linear)/2
  Bus Selector3/2 -> Single Track Model (linear)/3
  Bus Selector3/3 -> Single Track Model (linear)/4
  Bus Selector3/4 -> Single Track Model (linear)/5
  Bus Selector3/5 -> Single Track Model (linear)/6
  Bus Selector3/6 -> Single Track Model (linear)/7
  Demux/1 -> Single Track Model (linear)/9
  Demux/2 -> Single Track Model (linear)/10
  Demux/3 -> Single Track Model (linear)/11
  Demux/4 -> Single Track Model (linear)/12
  Demux/5 -> Single Track Model (linear)/13
  Demux/6 -> Single Track Model (linear)/14
  Demux/7 -> Single Track Model (linear)/15

== system SLlib_lka_thesis/Vehicle Models ext./Steering Model (CarMaker DSR) [Parameter; masked] ==
  Bus Creator2 : BusCreator  Inputs=9
  Constant1 : Constant  Value=i_HR
  Constant11 : Constant  Value=d_rot
  Constant13 : Constant  Value=m_right
  Constant14 : Constant  Value=m_left
  Constant15 : Constant  Value=I_rot
  Constant16 : Constant  Value=m_rack
  Constant17 : Constant  Value=V
  Constant18 : Constant  Value=alpha
  Constant4 : Constant  Value=d_rack
  SteerMdl_Parameter : Outport
  wires:
  Constant11/1 -> Bus Creator2/1  "d_rot"
  Constant4/1 -> Bus Creator2/2  "d_rack"
  Constant1/1 -> Bus Creator2/3  "i_HR"
  Constant15/1 -> Bus Creator2/4  "I_rot"
  Constant14/1 -> Bus Creator2/5  "m_left"
  Constant13/1 -> Bus Creator2/6  "m_right"
  Constant16/1 -> Bus Creator2/7  "m_rack"
  Constant17/1 -> Bus Creator2/8  "V"
  Constant18/1 -> Bus Creator2/9  "alpha"
  Bus Creator2/1 -> SteerMdl_Parameter/1

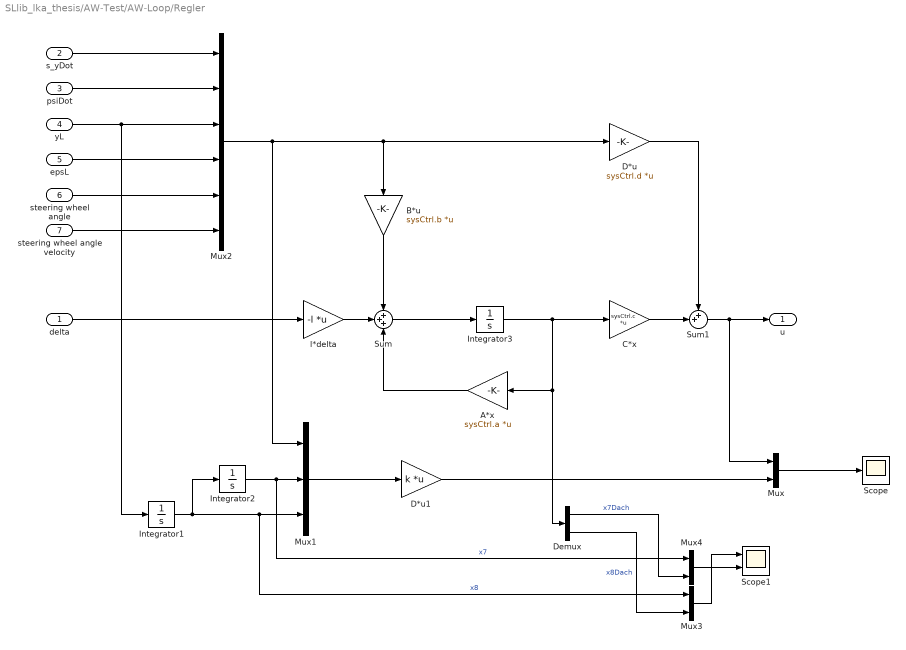
== system SLlib_lka_thesis/AW-Test/AW-Loop/Regler ==
  delta : Inport
  s_yDot : Inport  Port=2
  psiDot : Inport  Port=3
  yL : Inport  Port=4
  epsL : Inport  Port=5
  steering wheel angle : Inport  Port=6
  steering wheel angle velocity : Inport  Port=7
  A*x : Gain  Gain=sysCtrl.a  Multiplication=Matrix(K*u)
  B*u : Gain  Gain=sysCtrl.b  Multiplication=Matrix(K*u)
  C*x : Gain  Gain=sysCtrl.c  Multiplication=Matrix(K*u)
  D*u : Gain  Gain=sysCtrl.d  Multiplication=Matrix(K*u)
  D*u1 : Gain  Gain=k  Multiplication=Matrix(K*u)
  Demux : Demux  Outputs=2
  Integrator1 : Integrator
  Integrator2 : Integrator
  Integrator3 : Integrator
  Mux : Mux  Inputs=2
  Mux1 : Mux  Inputs=3
  Mux2 : Mux  Inputs=6
  Mux3 : Mux  Inputs=2
  Mux4 : Mux  Inputs=2
  Scope : Scope
  Scope1 : Scope  NumInputPorts=2
  Sum : Sum  Inputs=+++
  Sum1 : Sum  Inputs=++|
  l*delta : Gain  Gain=-l  Multiplication=Matrix(K*u)
  u : Outport
  wires:
  Mux4/1 -> Scope1/2
  Mux3/1 -> Scope1/1
  Demux/1 -> Mux4/2  "x7Dach"
  Demux/2 -> Mux3/2  "x8Dach"
  Mux/1 -> Scope/1
  D*u1/1 -> Mux/2
  Mux1/1 -> D*u1/1
  Integrator2/1 -> Mux4/1, Mux1/2  "x7"
  Integrator1/1 -> Mux3/1, Mux1/3, Integrator2/1  "x8"
  Sum1/1 -> Mux/1, u/1
  B*u/1 -> Sum/1
  D*u/1 -> Sum1/1
  C*x/1 -> Sum1/2
  delta/1 -> l*delta/1
  l*delta/1 -> Sum/2
  Mux2/1 -> Mux1/1, B*u/1, D*u/1
  steering wheel angle velocity/1 -> Mux2/6
  steering wheel angle/1 -> Mux2/5
  epsL/1 -> Mux2/4
  yL/1 -> Integrator1/1, Mux2/3
  psiDot/1 -> Mux2/2
  s_yDot/1 -> Mux2/1
  Sum/1 -> Integrator3/1
  Integrator3/1 -> Demux/1, A*x/1, C*x/1
  A*x/1 -> Sum/3

== system SLlib_lka_thesis/AW-Test/AW-Loop/Vehicle Model ==
  SWTorque [Nm] : Inport
  F_left [N] : Inport  Port=2
  curvature_LAD [1/m] : Inport  Port=3
  Bus Selector5 : BusSelector  OutputSignals=latOff_LAD_nonlinear
  Constant1 : Constant  Value=0
  Constant14 : Constant  Value=0
  Constant18 : Constant  Value=pin.L
  Constant19 : Constant  Value=pin.vx
  Gain1 : Gain  Gain=-1
  Single Track Model (linear) [Initial Values; masked] : $bdroot/Vehicle Models ext./Single Track Model (linear) [Initial Values; masked]  sy=0  vy=0  yawAngle=0  yawRate=0  x_global=0  y_global=0  s_global=0
  Single Track Model/LaneTracking/Steering Model : $bdroot/Vehicle Models ext./Single Track Model//Lane Tracking//Steering Model
  VehicleStates : Outport
  wires:
  F_left [N]/1 -> Gain1/1, Single Track Model/LaneTracking/Steering Model/7
  Constant14/1 -> Single Track Model/LaneTracking/Steering Model/10
  Constant19/1 -> Single Track Model/LaneTracking/Steering Model/4
  Constant18/1 -> Single Track Model/LaneTracking/Steering Model/5
  [VhclParam] -> Single Track Model/LaneTracking/Steering Model/2
  [SteerParam] -> Single Track Model/LaneTracking/Steering Model/3
  Single Track Model/LaneTracking/Steering Model/1 -> VehicleStates/1, Bus Selector5/1
  Bus Selector5/1 -> Single Track Model/LaneTracking/Steering Model/11  "<latOff_LAD_nonlinear>"
  SWTorque [Nm]/1 -> Single Track Model/LaneTracking/Steering Model/1
  Constant1/1 -> Single Track Model/LaneTracking/Steering Model/9
  Gain1/1 -> Single Track Model/LaneTracking/Steering Model/8
  curvature_LAD [1/m]/1 -> Single Track Model/LaneTracking/Steering Model/6
  Single Track Model (linear) [Initial Values; masked]/1 -> ?

== system SLlib_lka_thesis/LKA-Controller/AlgSynth/Controller ==
  r : Inport
  y : Inport  Port=2
  Gain : Gain  Gain=contr.s.AlgSynth.R.ss.a  Multiplication=Matrix(K*u) (u vector)
  Gain1 : Gain  Gain=-1
  Gain2 : Gain  Gain=contr.s.AlgSynth.R.ss.b
  Gain3 : Gain  Gain=contr.s.AlgSynth.V.ss.b
  Gain4 : Gain  Gain=contr.s.AlgSynth.V.ss.d
  Gain5 : Gain  Gain=contr.s.AlgSynth.R.ss.d
  Gain7 : Gain  Gain=contr.s.AlgSynth.R.ss.c  Multiplication=Matrix(K*u) (u vector)
  Integrator : Integrator
  Sum : Sum  Inputs=+++
  Sum1 : Sum  Inputs=+++
  u : Outport
  wires:
  Sum1/1 -> u/1
  Gain5/1 -> Sum1/3
  Gain4/1 -> Sum1/1
  Integrator/1 -> Gain/1, Gain7/1
  Gain3/1 -> Sum/1
  r/1 -> Gain4/1, Gain3/1
  Gain2/1 -> Sum/2
  Gain1/1 -> Gain5/1, Gain2/1  "-y"
  y/1 -> Gain1/1
  Sum/1 -> Integrator/1
  Gain/1 -> Sum/3
  Gain7/1 -> Sum1/2

== system SLlib_lka_thesis/Lane Tracking/Lane Tracking Sensor/Interface Lane Sensor ==
  note: Define bus signal names here!
  LAD [m] : Inport  OutDataTypeStr=double
  isValid_LAD [-] : Inport  Port=2  OutDataTypeStr=boolean
  lateralOff_LAD [m] : Inport  Port=3  OutDataTypeStr=double
  angularDev_LAD [rad] : Inport  Port=4  OutDataTypeStr=double
  roadCurv_LAD [1/m] : Inport  Port=5  OutDataTypeStr=double
  poly_lateralOff_LAD [m] : Inport  Port=6  OutDataTypeStr=double
  poly_angularDev_LAD [rad] : Inport  Port=7  OutDataTypeStr=double
  poly_roadCurvat_LAD [1/m] : Inport  Port=8  OutDataTypeStr=double
  poly_domain_LAD [1/m] : Inport  Port=9  OutDataTypeStr=double  PortDimensions=[2,1]
  Bus Creator : BusCreator  Inputs=9
  LaneSensor : Outport
  wires:
  poly_domain_LAD [1/m]/1 -> Bus Creator/9  "poly_domain_LAD_Sensor"
  poly_roadCurvat_LAD [1/m]/1 -> Bus Creator/8  "poly_roadCurvat_LAD_Sensor"
  poly_angularDev_LAD [rad]/1 -> Bus Creator/7  "poly_angularDev_LAD_Sensor"
  poly_lateralOff_LAD [m]/1 -> Bus Creator/6  "poly_lateralOff_LAD_Sensor"
  LAD [m]/1 -> Bus Creator/1  "LAD_Sensor"
  isValid_LAD [-]/1 -> Bus Creator/2  "isValid_LAD_Sensor"
  lateralOff_LAD [m]/1 -> Bus Creator/3  "lateralOff_LAD_Sensor"
  angularDev_LAD [rad]/1 -> Bus Creator/4  "angularDev_LAD_Sensor"
  roadCurv_LAD [1/m]/1 -> Bus Creator/5  "curvature_LAD_Sensor"
  Bus Creator/1 -> LaneSensor/1
